simulink library "helperlibrary"  (R2019b)
settings: Solver=VariableStepAuto  StartTime=0.0  StopTime=10.0  RelTol=1e-3
libraries: $bdroot x5

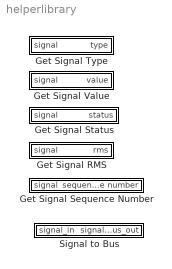
== system helperlibrary ==
  Get Signal RMS : Subsystem  TreatAsAtomicUnit=on
  Get Signal Sequence Number : Subsystem  TreatAsAtomicUnit=on
  Get Signal Status : Subsystem  TreatAsAtomicUnit=on
  Get Signal Type : Subsystem  TreatAsAtomicUnit=on
  Get Signal Value : Subsystem  TreatAsAtomicUnit=on
  Signal to Bus : Subsystem  TreatAsAtomicUnit=on

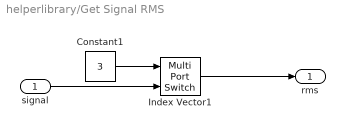
== system helperlibrary/Get Signal RMS ==
  signal : Inport
  Constant1 : Constant  Value=3
  Index Vector1 : MultiPortSwitch  DataPortOrder=Zero-based contiguous  Inputs=1  zeroidx=on
  rms : Outport
  wires:
  signal/1 -> Index Vector1/2
  Constant1/1 -> Index Vector1/1
  Index Vector1/1 -> rms/1

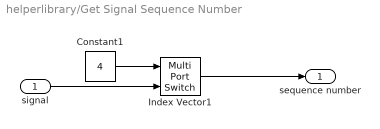
== system helperlibrary/Get Signal Sequence Number ==
  signal : Inport
  Constant1 : Constant  Value=4
  Index Vector1 : MultiPortSwitch  DataPortOrder=Zero-based contiguous  Inputs=1  zeroidx=on
  sequence number : Outport
  wires:
  Index Vector1/1 -> sequence number/1
  Constant1/1 -> Index Vector1/1
  signal/1 -> Index Vector1/2

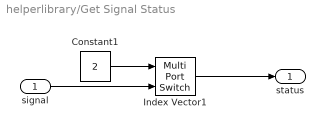
== system helperlibrary/Get Signal Status ==
  signal : Inport
  Constant1 : Constant  Value=2
  Index Vector1 : MultiPortSwitch  DataPortOrder=Zero-based contiguous  Inputs=1  zeroidx=on
  status : Outport
  wires:
  Constant1/1 -> Index Vector1/1
  signal/1 -> Index Vector1/2
  Index Vector1/1 -> status/1

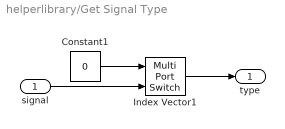
== system helperlibrary/Get Signal Type ==
  signal : Inport
  Constant1 : Constant  Value=0
  Index Vector1 : MultiPortSwitch  DataPortOrder=Zero-based contiguous  Inputs=1  zeroidx=on
  type : Outport
  wires:
  signal/1 -> Index Vector1/2
  Index Vector1/1 -> type/1
  Constant1/1 -> Index Vector1/1

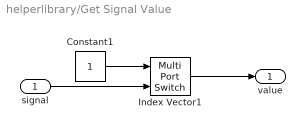
== system helperlibrary/Get Signal Value ==
  signal : Inport
  Constant1 : Constant
  Index Vector1 : MultiPortSwitch  DataPortOrder=Zero-based contiguous  Inputs=1  zeroidx=on
  value : Outport
  wires:
  Constant1/1 -> Index Vector1/1
  Index Vector1/1 -> value/1
  signal/1 -> Index Vector1/2

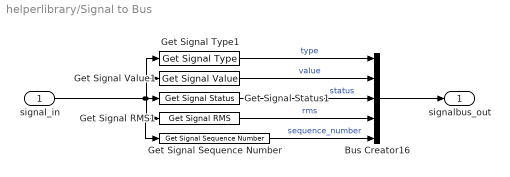
== system helperlibrary/Signal to Bus ==
  signal_in : Inport
  Bus Creator16 : BusCreator  Inputs=5
  Get Signal RMS1 : $bdroot/Get Signal RMS  SystemSampleTime=-1  Latency=0  AutoFrameSizeCalculation=off
  Get Signal Sequence Number : $bdroot/Get Signal Sequence Number  SystemSampleTime=-1  Latency=0  AutoFrameSizeCalculation=off
  Get Signal Status1 : $bdroot/Get Signal Status  SystemSampleTime=-1  Latency=0  AutoFrameSizeCalculation=off
  Get Signal Type1 : $bdroot/Get Signal Type  SystemSampleTime=-1  Latency=0  AutoFrameSizeCalculation=off
  Get Signal Value1 : $bdroot/Get Signal Value  SystemSampleTime=-1  Latency=0  AutoFrameSizeCalculation=off
  signalbus_out : Outport
  wires:
  Get Signal Value1/1 -> Bus Creator16/2  "value"
  Get Signal Status1/1 -> Bus Creator16/3  "status"
  Bus Creator16/1 -> signalbus_out/1
  signal_in/1 -> Get Signal Type1/1, Get Signal Value1/1, Get Signal Sequence Number/1, Get Signal RMS1/1, Get Signal Status1/1
  Get Signal Type1/1 -> Bus Creator16/1  "type"
  Get Signal RMS1/1 -> Bus Creator16/4  "rms"
  Get Signal Sequence Number/1 -> Bus Creator16/5  "sequence_number"
